simulink model "parallel_phase_voltages_per_switching_state_6"  (R2022a)
settings: Solver=FixedStepDiscrete  StartTime=0.0  StopTime=10.0  RelTol=1e-3
values from neighbouring files (symbols this model uses):
  f_c = 100000    [MPC_params.m]
  Rt = 1e-8    (= 1e-08)    [MPC_params.m]
  u_dc = 565    [MPC_params.m]
libraries: simulink x2, hdlsllib x2
(part 3 of 4)

== matlab function parallel_phase_voltages_per_switching_state_6/Phase_voltages_per_switching_state/Subsystem/MATLAB Function12 ==
  data: theta_el_with_offset input; d_voltage_per_switching_state output; u_dc_link_voltage input; Index input; q_voltage_per_switching_state output; x_voltage_per_switching_state output; y_voltage_per_switching_state output
function [d_voltage_per_switching_state, q_voltage_per_switching_state, x_voltage_per_switching_state, y_voltage_per_switching_state] = fcn(theta_el_with_offset, u_dc_link_voltage, Index)
      
        % Initial condition
            Index = Index+1+12;

    
        % Swichtingstates factors alpha beta x y
        Factors_alpha_beta_x_y = single([0	    0.333333333333333	-0.166666666666667	 0.166666666666667	-0.166666666666667	 0.166666666666667	-0.333333333333333	0	 0.288675134594813	0.622008467928146	 0.122008467928146  	0.455341801261480	 0.122008467928146	 0.455341801261480	-0.0446581987385205  0.288675134594813	-0.288675134594813	0.0446581987385205	-0.455341801261480	-0.122008467928146	-0.455341801261480	-0.122008467928146	-0.622008467928146	-0.288675134594813	0	                0.333333333333333	-0.166666666666667  	0.166666666666667	-0.166666666666667	 0.166666666666667	 -0.333333333333333	0	                 0	                 0.333333333333333	-0.166666666666667	  0.166666666666667	    -0.166666666666667	  0.166666666666667	    -0.333333333333333	 0	                 0.288675134594813	 0.622008467928146	 0.122008467928146	 0.455341801261480	 0.122008467928146	 0.455341801261480	-0.0446581987385205  0.288675134594813	-0.288675134594813	 0.0446581987385205  -0.455341801261480	  -0.122008467928146	-0.455341801261480	-0.122008467928146	-0.622008467928146	-0.288675134594813	0	0.333333333333333	-0.166666666666667	 0.166666666666667	-0.166666666666667	 0.166666666666667	-0.333333333333333	0;
                                         0	    0                    0.288675134594813	 0.288675134594813	-0.288675134594813	-0.288675134594813	 0	                0	 0.166666666666667	0.166666666666667	 0.455341801261480  	0.455341801261480	-0.122008467928146	-0.122008467928146	 0.166666666666667	 0.166666666666667	 0.166666666666667	0.166666666666667	 0.455341801261480   0.455341801261480	-0.122008467928146	-0.122008467928146	 0.166666666666667	 0.166666666666667	0.333333333333333	0.333333333333333	 0.622008467928146	    0.622008467928146	 0.0446581987385205	 0.0446581987385205	  0.333333333333333	0.333333333333333	-0.333333333333333	-0.333333333333333	-0.0446581987385205	 -0.0446581987385205	-0.622008467928146	 -0.622008467928146	    -0.333333333333333	-0.333333333333333	-0.166666666666667	-0.166666666666667	 0.122008467928146	 0.122008467928146	-0.455341801261480	-0.455341801261480	-0.166666666666667	-0.166666666666667	-0.166666666666667	-0.166666666666667	  0.122008467928146	   0.122008467928146	-0.455341801261480	-0.455341801261480	-0.166666666666667	-0.166666666666667	0	0	                 0.288675134594813	 0.288675134594813	-0.288675134594813	-0.288675134594813	 0	                0;
                                         0	    0.333333333333333	-0.166666666666667	 0.166666666666667	-0.166666666666667	 0.166666666666667	-0.333333333333333	0	-0.288675134594813	0.0446581987385205	-0.455341801261480	   -0.122008467928146	-0.455341801261480	-0.122008467928146	-0.622008467928146	-0.288675134594813	 0.288675134594813	0.622008467928146	 0.122008467928146	 0.455341801261480   0.122008467928146	 0.455341801261480	-0.0446581987385205	 0.288675134594813	0	                0.333333333333333	-0.166666666666667	    0.166666666666667	-0.166666666666667	 0.166666666666667	 -0.333333333333333	0	                 0	                 0.333333333333333	-0.166666666666667	  0.166666666666667	    -0.166666666666667	  0.166666666666667	    -0.333333333333333	 0	                -0.288675134594813	 0.0446581987385205	-0.455341801261480	-0.122008467928146	-0.455341801261480	-0.122008467928146	-0.622008467928146	-0.288675134594813	 0.288675134594813	 0.622008467928146	  0.122008467928146	   0.455341801261480	 0.122008467928146	 0.455341801261480	-0.0446581987385205  0.288675134594813	0	0.333333333333333	-0.166666666666667	 0.166666666666667	-0.166666666666667	 0.166666666666667	-0.333333333333333	0;
                                         0	    0	                -0.288675134594813	-0.288675134594813	 0.288675134594813	 0.288675134594813	 0              	0	 0.166666666666667	0.166666666666667	-0.122008467928146     -0.122008467928146	 0.455341801261480	 0.455341801261480	 0.166666666666667	 0.166666666666667	 0.166666666666667	0.166666666666667	-0.122008467928146	-0.122008467928146	 0.455341801261480	 0.455341801261480	 0.166666666666667	 0.166666666666667	0.333333333333333	0.333333333333333	 0.0446581987385205 	0.0446581987385205	 0.622008467928146	 0.622008467928146	  0.333333333333333	0.333333333333333	-0.333333333333333	-0.333333333333333	-0.622008467928146	 -0.622008467928146	    -0.0446581987385205	 -0.0446581987385205	-0.333333333333333	-0.333333333333333	-0.166666666666667	-0.166666666666667	-0.455341801261480	-0.455341801261480	 0.122008467928146	 0.122008467928146	-0.166666666666667	-0.166666666666667	-0.166666666666667	-0.166666666666667	 -0.455341801261480	  -0.455341801261480	 0.122008467928146	 0.122008467928146	-0.166666666666667	-0.166666666666667	0	0	                -0.288675134594813	-0.288675134594813	 0.288675134594813	 0.288675134594813	 0	                0]);
        
        % Park-Transformation of the switchingstates factors
        Factors_d_q_x_y =single(zeros(4,1));
    
        Factors_d_q_x_y(3,1) = Factors_alpha_beta_x_y(3,Index);
        Factors_d_q_x_y(4,1) = Factors_alpha_beta_x_y(4,Index);
    
        cos_theta_el = single(cos(theta_el_with_offset));
        sin_theta_el = single(sin(theta_el_with_offset));
       
        Factors_d_q_x_y(1,1) = cos_theta_el*Factors_alpha_beta_x_y(1,Index)+sin_theta_el*Factors_alpha_beta_x_y(2,Index);
        Factors_d_q_x_y(2,1) = -sin_theta_el*Factors_alpha_beta_x_y(1,Index)+cos_theta_el*Factors_alpha_beta_x_y(2,Index);
    
        %Calculation of the voltages per switching state in alpha beta coordinates
        d_q_x_y_voltages_per_switching_state = single(u_dc_link_voltage*Factors_d_q_x_y);
    
        d_voltage_per_switching_state = d_q_x_y_voltages_per_switching_state(1,1);
        q_voltage_per_switching_state = d_q_x_y_voltages_per_switching_state(2,1);
        x_voltage_per_switching_state = d_q_x_y_voltages_per_switching_state(3,1);
        y_voltage_per_switching_state = d_q_x_y_voltages_per_switching_state(4,1);
    

end

== matlab function parallel_phase_voltages_per_switching_state_6/Phase_voltages_per_switching_state/Subsystem/MATLAB Function13 ==
  data: theta_el_with_offset input; d_voltage_per_switching_state output; u_dc_link_voltage input; Index input; q_voltage_per_switching_state output; x_voltage_per_switching_state output; y_voltage_per_switching_state output
function [d_voltage_per_switching_state, q_voltage_per_switching_state, x_voltage_per_switching_state, y_voltage_per_switching_state] = fcn(theta_el_with_offset, u_dc_link_voltage, Index)
      
        % Initial condition
            Index = Index+1+8;

    
        % Swichtingstates factors alpha beta x y
        Factors_alpha_beta_x_y = single([0	    0.333333333333333	-0.166666666666667	 0.166666666666667	-0.166666666666667	 0.166666666666667	-0.333333333333333	0	 0.288675134594813	0.622008467928146	 0.122008467928146  	0.455341801261480	 0.122008467928146	 0.455341801261480	-0.0446581987385205  0.288675134594813	-0.288675134594813	0.0446581987385205	-0.455341801261480	-0.122008467928146	-0.455341801261480	-0.122008467928146	-0.622008467928146	-0.288675134594813	0	                0.333333333333333	-0.166666666666667  	0.166666666666667	-0.166666666666667	 0.166666666666667	 -0.333333333333333	0	                 0	                 0.333333333333333	-0.166666666666667	  0.166666666666667	    -0.166666666666667	  0.166666666666667	    -0.333333333333333	 0	                 0.288675134594813	 0.622008467928146	 0.122008467928146	 0.455341801261480	 0.122008467928146	 0.455341801261480	-0.0446581987385205  0.288675134594813	-0.288675134594813	 0.0446581987385205  -0.455341801261480	  -0.122008467928146	-0.455341801261480	-0.122008467928146	-0.622008467928146	-0.288675134594813	0	0.333333333333333	-0.166666666666667	 0.166666666666667	-0.166666666666667	 0.166666666666667	-0.333333333333333	0;
                                         0	    0                    0.288675134594813	 0.288675134594813	-0.288675134594813	-0.288675134594813	 0	                0	 0.166666666666667	0.166666666666667	 0.455341801261480  	0.455341801261480	-0.122008467928146	-0.122008467928146	 0.166666666666667	 0.166666666666667	 0.166666666666667	0.166666666666667	 0.455341801261480   0.455341801261480	-0.122008467928146	-0.122008467928146	 0.166666666666667	 0.166666666666667	0.333333333333333	0.333333333333333	 0.622008467928146	    0.622008467928146	 0.0446581987385205	 0.0446581987385205	  0.333333333333333	0.333333333333333	-0.333333333333333	-0.333333333333333	-0.0446581987385205	 -0.0446581987385205	-0.622008467928146	 -0.622008467928146	    -0.333333333333333	-0.333333333333333	-0.166666666666667	-0.166666666666667	 0.122008467928146	 0.122008467928146	-0.455341801261480	-0.455341801261480	-0.166666666666667	-0.166666666666667	-0.166666666666667	-0.166666666666667	  0.122008467928146	   0.122008467928146	-0.455341801261480	-0.455341801261480	-0.166666666666667	-0.166666666666667	0	0	                 0.288675134594813	 0.288675134594813	-0.288675134594813	-0.288675134594813	 0	                0;
                                         0	    0.333333333333333	-0.166666666666667	 0.166666666666667	-0.166666666666667	 0.166666666666667	-0.333333333333333	0	-0.288675134594813	0.0446581987385205	-0.455341801261480	   -0.122008467928146	-0.455341801261480	-0.122008467928146	-0.622008467928146	-0.288675134594813	 0.288675134594813	0.622008467928146	 0.122008467928146	 0.455341801261480   0.122008467928146	 0.455341801261480	-0.0446581987385205	 0.288675134594813	0	                0.333333333333333	-0.166666666666667	    0.166666666666667	-0.166666666666667	 0.166666666666667	 -0.333333333333333	0	                 0	                 0.333333333333333	-0.166666666666667	  0.166666666666667	    -0.166666666666667	  0.166666666666667	    -0.333333333333333	 0	                -0.288675134594813	 0.0446581987385205	-0.455341801261480	-0.122008467928146	-0.455341801261480	-0.122008467928146	-0.622008467928146	-0.288675134594813	 0.288675134594813	 0.622008467928146	  0.122008467928146	   0.455341801261480	 0.122008467928146	 0.455341801261480	-0.0446581987385205  0.288675134594813	0	0.333333333333333	-0.166666666666667	 0.166666666666667	-0.166666666666667	 0.166666666666667	-0.333333333333333	0;
                                         0	    0	                -0.288675134594813	-0.288675134594813	 0.288675134594813	 0.288675134594813	 0              	0	 0.166666666666667	0.166666666666667	-0.122008467928146     -0.122008467928146	 0.455341801261480	 0.455341801261480	 0.166666666666667	 0.166666666666667	 0.166666666666667	0.166666666666667	-0.122008467928146	-0.122008467928146	 0.455341801261480	 0.455341801261480	 0.166666666666667	 0.166666666666667	0.333333333333333	0.333333333333333	 0.0446581987385205 	0.0446581987385205	 0.622008467928146	 0.622008467928146	  0.333333333333333	0.333333333333333	-0.333333333333333	-0.333333333333333	-0.622008467928146	 -0.622008467928146	    -0.0446581987385205	 -0.0446581987385205	-0.333333333333333	-0.333333333333333	-0.166666666666667	-0.166666666666667	-0.455341801261480	-0.455341801261480	 0.122008467928146	 0.122008467928146	-0.166666666666667	-0.166666666666667	-0.166666666666667	-0.166666666666667	 -0.455341801261480	  -0.455341801261480	 0.122008467928146	 0.122008467928146	-0.166666666666667	-0.166666666666667	0	0	                -0.288675134594813	-0.288675134594813	 0.288675134594813	 0.288675134594813	 0	                0]);
        
        % Park-Transformation of the switchingstates factors
        Factors_d_q_x_y =single(zeros(4,1));
    
        Factors_d_q_x_y(3,1) = Factors_alpha_beta_x_y(3,Index);
        Factors_d_q_x_y(4,1) = Factors_alpha_beta_x_y(4,Index);
    
        cos_theta_el = single(cos(theta_el_with_offset));
        sin_theta_el = single(sin(theta_el_with_offset));
       
        Factors_d_q_x_y(1,1) = cos_theta_el*Factors_alpha_beta_x_y(1,Index)+sin_theta_el*Factors_alpha_beta_x_y(2,Index);
        Factors_d_q_x_y(2,1) = -sin_theta_el*Factors_alpha_beta_x_y(1,Index)+cos_theta_el*Factors_alpha_beta_x_y(2,Index);
    
        %Calculation of the voltages per switching state in alpha beta coordinates
        d_q_x_y_voltages_per_switching_state = single(u_dc_link_voltage*Factors_d_q_x_y);
    
        d_voltage_per_switching_state = d_q_x_y_voltages_per_switching_state(1,1);
        q_voltage_per_switching_state = d_q_x_y_voltages_per_switching_state(2,1);
        x_voltage_per_switching_state = d_q_x_y_voltages_per_switching_state(3,1);
        y_voltage_per_switching_state = d_q_x_y_voltages_per_switching_state(4,1);
    

end

== matlab function parallel_phase_voltages_per_switching_state_6/Phase_voltages_per_switching_state/Subsystem/MATLAB Function14 ==
  data: theta_el_with_offset input; d_voltage_per_switching_state output; u_dc_link_voltage input; Index input; q_voltage_per_switching_state output; x_voltage_per_switching_state output; y_voltage_per_switching_state output
function [d_voltage_per_switching_state, q_voltage_per_switching_state, x_voltage_per_switching_state, y_voltage_per_switching_state] = fcn(theta_el_with_offset, u_dc_link_voltage, Index)
      
        % Initial condition
            Index = Index+1+4;

    
        % Swichtingstates factors alpha beta x y
        Factors_alpha_beta_x_y = single([0	    0.333333333333333	-0.166666666666667	 0.166666666666667	-0.166666666666667	 0.166666666666667	-0.333333333333333	0	 0.288675134594813	0.622008467928146	 0.122008467928146  	0.455341801261480	 0.122008467928146	 0.455341801261480	-0.0446581987385205  0.288675134594813	-0.288675134594813	0.0446581987385205	-0.455341801261480	-0.122008467928146	-0.455341801261480	-0.122008467928146	-0.622008467928146	-0.288675134594813	0	                0.333333333333333	-0.166666666666667  	0.166666666666667	-0.166666666666667	 0.166666666666667	 -0.333333333333333	0	                 0	                 0.333333333333333	-0.166666666666667	  0.166666666666667	    -0.166666666666667	  0.166666666666667	    -0.333333333333333	 0	                 0.288675134594813	 0.622008467928146	 0.122008467928146	 0.455341801261480	 0.122008467928146	 0.455341801261480	-0.0446581987385205  0.288675134594813	-0.288675134594813	 0.0446581987385205  -0.455341801261480	  -0.122008467928146	-0.455341801261480	-0.122008467928146	-0.622008467928146	-0.288675134594813	0	0.333333333333333	-0.166666666666667	 0.166666666666667	-0.166666666666667	 0.166666666666667	-0.333333333333333	0;
                                         0	    0                    0.288675134594813	 0.288675134594813	-0.288675134594813	-0.288675134594813	 0	                0	 0.166666666666667	0.166666666666667	 0.455341801261480  	0.455341801261480	-0.122008467928146	-0.122008467928146	 0.166666666666667	 0.166666666666667	 0.166666666666667	0.166666666666667	 0.455341801261480   0.455341801261480	-0.122008467928146	-0.122008467928146	 0.166666666666667	 0.166666666666667	0.333333333333333	0.333333333333333	 0.622008467928146	    0.622008467928146	 0.0446581987385205	 0.0446581987385205	  0.333333333333333	0.333333333333333	-0.333333333333333	-0.333333333333333	-0.0446581987385205	 -0.0446581987385205	-0.622008467928146	 -0.622008467928146	    -0.333333333333333	-0.333333333333333	-0.166666666666667	-0.166666666666667	 0.122008467928146	 0.122008467928146	-0.455341801261480	-0.455341801261480	-0.166666666666667	-0.166666666666667	-0.166666666666667	-0.166666666666667	  0.122008467928146	   0.122008467928146	-0.455341801261480	-0.455341801261480	-0.166666666666667	-0.166666666666667	0	0	                 0.288675134594813	 0.288675134594813	-0.288675134594813	-0.288675134594813	 0	                0;
                                         0	    0.333333333333333	-0.166666666666667	 0.166666666666667	-0.166666666666667	 0.166666666666667	-0.333333333333333	0	-0.288675134594813	0.0446581987385205	-0.455341801261480	   -0.122008467928146	-0.455341801261480	-0.122008467928146	-0.622008467928146	-0.288675134594813	 0.288675134594813	0.622008467928146	 0.122008467928146	 0.455341801261480   0.122008467928146	 0.455341801261480	-0.0446581987385205	 0.288675134594813	0	                0.333333333333333	-0.166666666666667	    0.166666666666667	-0.166666666666667	 0.166666666666667	 -0.333333333333333	0	                 0	                 0.333333333333333	-0.166666666666667	  0.166666666666667	    -0.166666666666667	  0.166666666666667	    -0.333333333333333	 0	                -0.288675134594813	 0.0446581987385205	-0.455341801261480	-0.122008467928146	-0.455341801261480	-0.122008467928146	-0.622008467928146	-0.288675134594813	 0.288675134594813	 0.622008467928146	  0.122008467928146	   0.455341801261480	 0.122008467928146	 0.455341801261480	-0.0446581987385205  0.288675134594813	0	0.333333333333333	-0.166666666666667	 0.166666666666667	-0.166666666666667	 0.166666666666667	-0.333333333333333	0;
                                         0	    0	                -0.288675134594813	-0.288675134594813	 0.288675134594813	 0.288675134594813	 0              	0	 0.166666666666667	0.166666666666667	-0.122008467928146     -0.122008467928146	 0.455341801261480	 0.455341801261480	 0.166666666666667	 0.166666666666667	 0.166666666666667	0.166666666666667	-0.122008467928146	-0.122008467928146	 0.455341801261480	 0.455341801261480	 0.166666666666667	 0.166666666666667	0.333333333333333	0.333333333333333	 0.0446581987385205 	0.0446581987385205	 0.622008467928146	 0.622008467928146	  0.333333333333333	0.333333333333333	-0.333333333333333	-0.333333333333333	-0.622008467928146	 -0.622008467928146	    -0.0446581987385205	 -0.0446581987385205	-0.333333333333333	-0.333333333333333	-0.166666666666667	-0.166666666666667	-0.455341801261480	-0.455341801261480	 0.122008467928146	 0.122008467928146	-0.166666666666667	-0.166666666666667	-0.166666666666667	-0.166666666666667	 -0.455341801261480	  -0.455341801261480	 0.122008467928146	 0.122008467928146	-0.166666666666667	-0.166666666666667	0	0	                -0.288675134594813	-0.288675134594813	 0.288675134594813	 0.288675134594813	 0	                0]);
        
        % Park-Transformation of the switchingstates factors
        Factors_d_q_x_y =single(zeros(4,1));
    
        Factors_d_q_x_y(3,1) = Factors_alpha_beta_x_y(3,Index);
        Factors_d_q_x_y(4,1) = Factors_alpha_beta_x_y(4,Index);
    
        cos_theta_el = single(cos(theta_el_with_offset));
        sin_theta_el = single(sin(theta_el_with_offset));
       
        Factors_d_q_x_y(1,1) = cos_theta_el*Factors_alpha_beta_x_y(1,Index)+sin_theta_el*Factors_alpha_beta_x_y(2,Index);
        Factors_d_q_x_y(2,1) = -sin_theta_el*Factors_alpha_beta_x_y(1,Index)+cos_theta_el*Factors_alpha_beta_x_y(2,Index);
    
        %Calculation of the voltages per switching state in alpha beta coordinates
        d_q_x_y_voltages_per_switching_state = single(u_dc_link_voltage*Factors_d_q_x_y);
    
        d_voltage_per_switching_state = d_q_x_y_voltages_per_switching_state(1,1);
        q_voltage_per_switching_state = d_q_x_y_voltages_per_switching_state(2,1);
        x_voltage_per_switching_state = d_q_x_y_voltages_per_switching_state(3,1);
        y_voltage_per_switching_state = d_q_x_y_voltages_per_switching_state(4,1);
    

end

== matlab function parallel_phase_voltages_per_switching_state_6/Phase_voltages_per_switching_state/Subsystem/MATLAB Function15 ==
  data: theta_el_with_offset input; d_voltage_per_switching_state output; u_dc_link_voltage input; Index input; q_voltage_per_switching_state output; x_voltage_per_switching_state output; y_voltage_per_switching_state output
function [d_voltage_per_switching_state, q_voltage_per_switching_state, x_voltage_per_switching_state, y_voltage_per_switching_state] = fcn(theta_el_with_offset, u_dc_link_voltage, Index)
      
        % Initial condition
            Index = Index+1;

        % Swichtingstates factors alpha beta x y
        Factors_alpha_beta_x_y = single([0	    0.333333333333333	-0.166666666666667	 0.166666666666667	-0.166666666666667	 0.166666666666667	-0.333333333333333	0	 0.288675134594813	0.622008467928146	 0.122008467928146  	0.455341801261480	 0.122008467928146	 0.455341801261480	-0.0446581987385205  0.288675134594813	-0.288675134594813	0.0446581987385205	-0.455341801261480	-0.122008467928146	-0.455341801261480	-0.122008467928146	-0.622008467928146	-0.288675134594813	0	                0.333333333333333	-0.166666666666667  	0.166666666666667	-0.166666666666667	 0.166666666666667	 -0.333333333333333	0	                 0	                 0.333333333333333	-0.166666666666667	  0.166666666666667	    -0.166666666666667	  0.166666666666667	    -0.333333333333333	 0	                 0.288675134594813	 0.622008467928146	 0.122008467928146	 0.455341801261480	 0.122008467928146	 0.455341801261480	-0.0446581987385205  0.288675134594813	-0.288675134594813	 0.0446581987385205  -0.455341801261480	  -0.122008467928146	-0.455341801261480	-0.122008467928146	-0.622008467928146	-0.288675134594813	0	0.333333333333333	-0.166666666666667	 0.166666666666667	-0.166666666666667	 0.166666666666667	-0.333333333333333	0;
                                         0	    0                    0.288675134594813	 0.288675134594813	-0.288675134594813	-0.288675134594813	 0	                0	 0.166666666666667	0.166666666666667	 0.455341801261480  	0.455341801261480	-0.122008467928146	-0.122008467928146	 0.166666666666667	 0.166666666666667	 0.166666666666667	0.166666666666667	 0.455341801261480   0.455341801261480	-0.122008467928146	-0.122008467928146	 0.166666666666667	 0.166666666666667	0.333333333333333	0.333333333333333	 0.622008467928146	    0.622008467928146	 0.0446581987385205	 0.0446581987385205	  0.333333333333333	0.333333333333333	-0.333333333333333	-0.333333333333333	-0.0446581987385205	 -0.0446581987385205	-0.622008467928146	 -0.622008467928146	    -0.333333333333333	-0.333333333333333	-0.166666666666667	-0.166666666666667	 0.122008467928146	 0.122008467928146	-0.455341801261480	-0.455341801261480	-0.166666666666667	-0.166666666666667	-0.166666666666667	-0.166666666666667	  0.122008467928146	   0.122008467928146	-0.455341801261480	-0.455341801261480	-0.166666666666667	-0.166666666666667	0	0	                 0.288675134594813	 0.288675134594813	-0.288675134594813	-0.288675134594813	 0	                0;
                                         0	    0.333333333333333	-0.166666666666667	 0.166666666666667	-0.166666666666667	 0.166666666666667	-0.333333333333333	0	-0.288675134594813	0.0446581987385205	-0.455341801261480	   -0.122008467928146	-0.455341801261480	-0.122008467928146	-0.622008467928146	-0.288675134594813	 0.288675134594813	0.622008467928146	 0.122008467928146	 0.455341801261480   0.122008467928146	 0.455341801261480	-0.0446581987385205	 0.288675134594813	0	                0.333333333333333	-0.166666666666667	    0.166666666666667	-0.166666666666667	 0.166666666666667	 -0.333333333333333	0	                 0	                 0.333333333333333	-0.166666666666667	  0.166666666666667	    -0.166666666666667	  0.166666666666667	    -0.333333333333333	 0	                -0.288675134594813	 0.0446581987385205	-0.455341801261480	-0.122008467928146	-0.455341801261480	-0.122008467928146	-0.622008467928146	-0.288675134594813	 0.288675134594813	 0.622008467928146	  0.122008467928146	   0.455341801261480	 0.122008467928146	 0.455341801261480	-0.0446581987385205  0.288675134594813	0	0.333333333333333	-0.166666666666667	 0.166666666666667	-0.166666666666667	 0.166666666666667	-0.333333333333333	0;
                                         0	    0	                -0.288675134594813	-0.288675134594813	 0.288675134594813	 0.288675134594813	 0              	0	 0.166666666666667	0.166666666666667	-0.122008467928146     -0.122008467928146	 0.455341801261480	 0.455341801261480	 0.166666666666667	 0.166666666666667	 0.166666666666667	0.166666666666667	-0.122008467928146	-0.122008467928146	 0.455341801261480	 0.455341801261480	 0.166666666666667	 0.166666666666667	0.333333333333333	0.333333333333333	 0.0446581987385205 	0.0446581987385205	 0.622008467928146	 0.622008467928146	  0.333333333333333	0.333333333333333	-0.333333333333333	-0.333333333333333	-0.622008467928146	 -0.622008467928146	    -0.0446581987385205	 -0.0446581987385205	-0.333333333333333	-0.333333333333333	-0.166666666666667	-0.166666666666667	-0.455341801261480	-0.455341801261480	 0.122008467928146	 0.122008467928146	-0.166666666666667	-0.166666666666667	-0.166666666666667	-0.166666666666667	 -0.455341801261480	  -0.455341801261480	 0.122008467928146	 0.122008467928146	-0.166666666666667	-0.166666666666667	0	0	                -0.288675134594813	-0.288675134594813	 0.288675134594813	 0.288675134594813	 0	                0]);
        
        % Park-Transformation of the switchingstates factors
        Factors_d_q_x_y =single(zeros(4,1));
    
        Factors_d_q_x_y(3,1) = Factors_alpha_beta_x_y(3,Index);
        Factors_d_q_x_y(4,1) = Factors_alpha_beta_x_y(4,Index);
    
        cos_theta_el = single(cos(theta_el_with_offset));
        sin_theta_el = single(sin(theta_el_with_offset));
       
        Factors_d_q_x_y(1,1) = cos_theta_el*Factors_alpha_beta_x_y(1,Index)+sin_theta_el*Factors_alpha_beta_x_y(2,Index);
        Factors_d_q_x_y(2,1) = -sin_theta_el*Factors_alpha_beta_x_y(1,Index)+cos_theta_el*Factors_alpha_beta_x_y(2,Index);
    
        %Calculation of the voltages per switching state in alpha beta coordinates
        d_q_x_y_voltages_per_switching_state = single(u_dc_link_voltage*Factors_d_q_x_y);
    
        d_voltage_per_switching_state = d_q_x_y_voltages_per_switching_state(1,1);
        q_voltage_per_switching_state = d_q_x_y_voltages_per_switching_state(2,1);
        x_voltage_per_switching_state = d_q_x_y_voltages_per_switching_state(3,1);
        y_voltage_per_switching_state = d_q_x_y_voltages_per_switching_state(4,1);
    

end

== matlab function parallel_phase_voltages_per_switching_state_6/Phase_voltages_per_switching_state/Subsystem/MATLAB Function1 ==
  data: theta_el_with_offset input; d_voltage_per_switching_state output; u_dc_link_voltage input; Index input; q_voltage_per_switching_state output; x_voltage_per_switching_state output; y_voltage_per_switching_state output
function [d_voltage_per_switching_state, q_voltage_per_switching_state, x_voltage_per_switching_state, y_voltage_per_switching_state] = fcn(theta_el_with_offset, u_dc_link_voltage, Index)
      
        % Initial condition
            Index = Index+1+56;

    
        % Swichtingstates factors alpha beta x y
        Factors_alpha_beta_x_y = single([0	    0.333333333333333	-0.166666666666667	 0.166666666666667	-0.166666666666667	 0.166666666666667	-0.333333333333333	0	 0.288675134594813	0.622008467928146	 0.122008467928146  	0.455341801261480	 0.122008467928146	 0.455341801261480	-0.0446581987385205  0.288675134594813	-0.288675134594813	0.0446581987385205	-0.455341801261480	-0.122008467928146	-0.455341801261480	-0.122008467928146	-0.622008467928146	-0.288675134594813	0	                0.333333333333333	-0.166666666666667  	0.166666666666667	-0.166666666666667	 0.166666666666667	 -0.333333333333333	0	                 0	                 0.333333333333333	-0.166666666666667	  0.166666666666667	    -0.166666666666667	  0.166666666666667	    -0.333333333333333	 0	                 0.288675134594813	 0.622008467928146	 0.122008467928146	 0.455341801261480	 0.122008467928146	 0.455341801261480	-0.0446581987385205  0.288675134594813	-0.288675134594813	 0.0446581987385205  -0.455341801261480	  -0.122008467928146	-0.455341801261480	-0.122008467928146	-0.622008467928146	-0.288675134594813	0	0.333333333333333	-0.166666666666667	 0.166666666666667	-0.166666666666667	 0.166666666666667	-0.333333333333333	0;
                                         0	    0                    0.288675134594813	 0.288675134594813	-0.288675134594813	-0.288675134594813	 0	                0	 0.166666666666667	0.166666666666667	 0.455341801261480  	0.455341801261480	-0.122008467928146	-0.122008467928146	 0.166666666666667	 0.166666666666667	 0.166666666666667	0.166666666666667	 0.455341801261480   0.455341801261480	-0.122008467928146	-0.122008467928146	 0.166666666666667	 0.166666666666667	0.333333333333333	0.333333333333333	 0.622008467928146	    0.622008467928146	 0.0446581987385205	 0.0446581987385205	  0.333333333333333	0.333333333333333	-0.333333333333333	-0.333333333333333	-0.0446581987385205	 -0.0446581987385205	-0.622008467928146	 -0.622008467928146	    -0.333333333333333	-0.333333333333333	-0.166666666666667	-0.166666666666667	 0.122008467928146	 0.122008467928146	-0.455341801261480	-0.455341801261480	-0.166666666666667	-0.166666666666667	-0.166666666666667	-0.166666666666667	  0.122008467928146	   0.122008467928146	-0.455341801261480	-0.455341801261480	-0.166666666666667	-0.166666666666667	0	0	                 0.288675134594813	 0.288675134594813	-0.288675134594813	-0.288675134594813	 0	                0;
                                         0	    0.333333333333333	-0.166666666666667	 0.166666666666667	-0.166666666666667	 0.166666666666667	-0.333333333333333	0	-0.288675134594813	0.0446581987385205	-0.455341801261480	   -0.122008467928146	-0.455341801261480	-0.122008467928146	-0.622008467928146	-0.288675134594813	 0.288675134594813	0.622008467928146	 0.122008467928146	 0.455341801261480   0.122008467928146	 0.455341801261480	-0.0446581987385205	 0.288675134594813	0	                0.333333333333333	-0.166666666666667	    0.166666666666667	-0.166666666666667	 0.166666666666667	 -0.333333333333333	0	                 0	                 0.333333333333333	-0.166666666666667	  0.166666666666667	    -0.166666666666667	  0.166666666666667	    -0.333333333333333	 0	                -0.288675134594813	 0.0446581987385205	-0.455341801261480	-0.122008467928146	-0.455341801261480	-0.122008467928146	-0.622008467928146	-0.288675134594813	 0.288675134594813	 0.622008467928146	  0.122008467928146	   0.455341801261480	 0.122008467928146	 0.455341801261480	-0.0446581987385205  0.288675134594813	0	0.333333333333333	-0.166666666666667	 0.166666666666667	-0.166666666666667	 0.166666666666667	-0.333333333333333	0;
                                         0	    0	                -0.288675134594813	-0.288675134594813	 0.288675134594813	 0.288675134594813	 0              	0	 0.166666666666667	0.166666666666667	-0.122008467928146     -0.122008467928146	 0.455341801261480	 0.455341801261480	 0.166666666666667	 0.166666666666667	 0.166666666666667	0.166666666666667	-0.122008467928146	-0.122008467928146	 0.455341801261480	 0.455341801261480	 0.166666666666667	 0.166666666666667	0.333333333333333	0.333333333333333	 0.0446581987385205 	0.0446581987385205	 0.622008467928146	 0.622008467928146	  0.333333333333333	0.333333333333333	-0.333333333333333	-0.333333333333333	-0.622008467928146	 -0.622008467928146	    -0.0446581987385205	 -0.0446581987385205	-0.333333333333333	-0.333333333333333	-0.166666666666667	-0.166666666666667	-0.455341801261480	-0.455341801261480	 0.122008467928146	 0.122008467928146	-0.166666666666667	-0.166666666666667	-0.166666666666667	-0.166666666666667	 -0.455341801261480	  -0.455341801261480	 0.122008467928146	 0.122008467928146	-0.166666666666667	-0.166666666666667	0	0	                -0.288675134594813	-0.288675134594813	 0.288675134594813	 0.288675134594813	 0	                0]);
        
        % Park-Transformation of the switchingstates factors
        Factors_d_q_x_y =single(zeros(4,1));
    
        Factors_d_q_x_y(3,1) = Factors_alpha_beta_x_y(3,Index);
        Factors_d_q_x_y(4,1) = Factors_alpha_beta_x_y(4,Index);
    
        cos_theta_el = single(cos(theta_el_with_offset));
        sin_theta_el = single(sin(theta_el_with_offset));
       
        Factors_d_q_x_y(1,1) = cos_theta_el*Factors_alpha_beta_x_y(1,Index)+sin_theta_el*Factors_alpha_beta_x_y(2,Index);
        Factors_d_q_x_y(2,1) = -sin_theta_el*Factors_alpha_beta_x_y(1,Index)+cos_theta_el*Factors_alpha_beta_x_y(2,Index);
    
        %Calculation of the voltages per switching state in alpha beta coordinates
        d_q_x_y_voltages_per_switching_state = single(u_dc_link_voltage*Factors_d_q_x_y);
    
        d_voltage_per_switching_state = d_q_x_y_voltages_per_switching_state(1,1);
        q_voltage_per_switching_state = d_q_x_y_voltages_per_switching_state(2,1);
        x_voltage_per_switching_state = d_q_x_y_voltages_per_switching_state(3,1);
        y_voltage_per_switching_state = d_q_x_y_voltages_per_switching_state(4,1);
    

end

== matlab function parallel_phase_voltages_per_switching_state_6/Phase_voltages_per_switching_state/Subsystem/MATLAB Function2 ==
  data: theta_el_with_offset input; d_voltage_per_switching_state output; u_dc_link_voltage input; Index input; q_voltage_per_switching_state output; x_voltage_per_switching_state output; y_voltage_per_switching_state output
function [d_voltage_per_switching_state, q_voltage_per_switching_state, x_voltage_per_switching_state, y_voltage_per_switching_state] = fcn(theta_el_with_offset, u_dc_link_voltage, Index)
      
        % Initial condition
            Index = Index+1+52;

        % Swichtingstates factors alpha beta x y
        Factors_alpha_beta_x_y = single([0	    0.333333333333333	-0.166666666666667	 0.166666666666667	-0.166666666666667	 0.166666666666667	-0.333333333333333	0	 0.288675134594813	0.622008467928146	 0.122008467928146  	0.455341801261480	 0.122008467928146	 0.455341801261480	-0.0446581987385205  0.288675134594813	-0.288675134594813	0.0446581987385205	-0.455341801261480	-0.122008467928146	-0.455341801261480	-0.122008467928146	-0.622008467928146	-0.288675134594813	0	                0.333333333333333	-0.166666666666667  	0.166666666666667	-0.166666666666667	 0.166666666666667	 -0.333333333333333	0	                 0	                 0.333333333333333	-0.166666666666667	  0.166666666666667	    -0.166666666666667	  0.166666666666667	    -0.333333333333333	 0	                 0.288675134594813	 0.622008467928146	 0.122008467928146	 0.455341801261480	 0.122008467928146	 0.455341801261480	-0.0446581987385205  0.288675134594813	-0.288675134594813	 0.0446581987385205  -0.455341801261480	  -0.122008467928146	-0.455341801261480	-0.122008467928146	-0.622008467928146	-0.288675134594813	0	0.333333333333333	-0.166666666666667	 0.166666666666667	-0.166666666666667	 0.166666666666667	-0.333333333333333	0;
                                         0	    0                    0.288675134594813	 0.288675134594813	-0.288675134594813	-0.288675134594813	 0	                0	 0.166666666666667	0.166666666666667	 0.455341801261480  	0.455341801261480	-0.122008467928146	-0.122008467928146	 0.166666666666667	 0.166666666666667	 0.166666666666667	0.166666666666667	 0.455341801261480   0.455341801261480	-0.122008467928146	-0.122008467928146	 0.166666666666667	 0.166666666666667	0.333333333333333	0.333333333333333	 0.622008467928146	    0.622008467928146	 0.0446581987385205	 0.0446581987385205	  0.333333333333333	0.333333333333333	-0.333333333333333	-0.333333333333333	-0.0446581987385205	 -0.0446581987385205	-0.622008467928146	 -0.622008467928146	    -0.333333333333333	-0.333333333333333	-0.166666666666667	-0.166666666666667	 0.122008467928146	 0.122008467928146	-0.455341801261480	-0.455341801261480	-0.166666666666667	-0.166666666666667	-0.166666666666667	-0.166666666666667	  0.122008467928146	   0.122008467928146	-0.455341801261480	-0.455341801261480	-0.166666666666667	-0.166666666666667	0	0	                 0.288675134594813	 0.288675134594813	-0.288675134594813	-0.288675134594813	 0	                0;
                                         0	    0.333333333333333	-0.166666666666667	 0.166666666666667	-0.166666666666667	 0.166666666666667	-0.333333333333333	0	-0.288675134594813	0.0446581987385205	-0.455341801261480	   -0.122008467928146	-0.455341801261480	-0.122008467928146	-0.622008467928146	-0.288675134594813	 0.288675134594813	0.622008467928146	 0.122008467928146	 0.455341801261480   0.122008467928146	 0.455341801261480	-0.0446581987385205	 0.288675134594813	0	                0.333333333333333	-0.166666666666667	    0.166666666666667	-0.166666666666667	 0.166666666666667	 -0.333333333333333	0	                 0	                 0.333333333333333	-0.166666666666667	  0.166666666666667	    -0.166666666666667	  0.166666666666667	    -0.333333333333333	 0	                -0.288675134594813	 0.0446581987385205	-0.455341801261480	-0.122008467928146	-0.455341801261480	-0.122008467928146	-0.622008467928146	-0.288675134594813	 0.288675134594813	 0.622008467928146	  0.122008467928146	   0.455341801261480	 0.122008467928146	 0.455341801261480	-0.0446581987385205  0.288675134594813	0	0.333333333333333	-0.166666666666667	 0.166666666666667	-0.166666666666667	 0.166666666666667	-0.333333333333333	0;
                                         0	    0	                -0.288675134594813	-0.288675134594813	 0.288675134594813	 0.288675134594813	 0              	0	 0.166666666666667	0.166666666666667	-0.122008467928146     -0.122008467928146	 0.455341801261480	 0.455341801261480	 0.166666666666667	 0.166666666666667	 0.166666666666667	0.166666666666667	-0.122008467928146	-0.122008467928146	 0.455341801261480	 0.455341801261480	 0.166666666666667	 0.166666666666667	0.333333333333333	0.333333333333333	 0.0446581987385205 	0.0446581987385205	 0.622008467928146	 0.622008467928146	  0.333333333333333	0.333333333333333	-0.333333333333333	-0.333333333333333	-0.622008467928146	 -0.622008467928146	    -0.0446581987385205	 -0.0446581987385205	-0.333333333333333	-0.333333333333333	-0.166666666666667	-0.166666666666667	-0.455341801261480	-0.455341801261480	 0.122008467928146	 0.122008467928146	-0.166666666666667	-0.166666666666667	-0.166666666666667	-0.166666666666667	 -0.455341801261480	  -0.455341801261480	 0.122008467928146	 0.122008467928146	-0.166666666666667	-0.166666666666667	0	0	                -0.288675134594813	-0.288675134594813	 0.288675134594813	 0.288675134594813	 0	                0]);
        
        % Park-Transformation of the switchingstates factors
        Factors_d_q_x_y =single(zeros(4,1));
    
        Factors_d_q_x_y(3,1) = Factors_alpha_beta_x_y(3,Index);
        Factors_d_q_x_y(4,1) = Factors_alpha_beta_x_y(4,Index);
    
        cos_theta_el = single(cos(theta_el_with_offset));
        sin_theta_el = single(sin(theta_el_with_offset));
       
        Factors_d_q_x_y(1,1) = cos_theta_el*Factors_alpha_beta_x_y(1,Index)+sin_theta_el*Factors_alpha_beta_x_y(2,Index);
        Factors_d_q_x_y(2,1) = -sin_theta_el*Factors_alpha_beta_x_y(1,Index)+cos_theta_el*Factors_alpha_beta_x_y(2,Index);
    
        %Calculation of the voltages per switching state in alpha beta coordinates
        d_q_x_y_voltages_per_switching_state = single(u_dc_link_voltage*Factors_d_q_x_y);
    
        d_voltage_per_switching_state = d_q_x_y_voltages_per_switching_state(1,1);
        q_voltage_per_switching_state = d_q_x_y_voltages_per_switching_state(2,1);
        x_voltage_per_switching_state = d_q_x_y_voltages_per_switching_state(3,1);
        y_voltage_per_switching_state = d_q_x_y_voltages_per_switching_state(4,1);
    

end

== matlab function parallel_phase_voltages_per_switching_state_6/Phase_voltages_per_switching_state/Subsystem/MATLAB Function3 ==
  data: theta_el_with_offset input; d_voltage_per_switching_state output; u_dc_link_voltage input; Index input; q_voltage_per_switching_state output; x_voltage_per_switching_state output; y_voltage_per_switching_state output
function [d_voltage_per_switching_state, q_voltage_per_switching_state, x_voltage_per_switching_state, y_voltage_per_switching_state] = fcn(theta_el_with_offset, u_dc_link_voltage, Index)
      
        % Initial condition
            Index = Index+1+48;

    
        % Swichtingstates factors alpha beta x y
        Factors_alpha_beta_x_y = single([0	    0.333333333333333	-0.166666666666667	 0.166666666666667	-0.166666666666667	 0.166666666666667	-0.333333333333333	0	 0.288675134594813	0.622008467928146	 0.122008467928146  	0.455341801261480	 0.122008467928146	 0.455341801261480	-0.0446581987385205  0.288675134594813	-0.288675134594813	0.0446581987385205	-0.455341801261480	-0.122008467928146	-0.455341801261480	-0.122008467928146	-0.622008467928146	-0.288675134594813	0	                0.333333333333333	-0.166666666666667  	0.166666666666667	-0.166666666666667	 0.166666666666667	 -0.333333333333333	0	                 0	                 0.333333333333333	-0.166666666666667	  0.166666666666667	    -0.166666666666667	  0.166666666666667	    -0.333333333333333	 0	                 0.288675134594813	 0.622008467928146	 0.122008467928146	 0.455341801261480	 0.122008467928146	 0.455341801261480	-0.0446581987385205  0.288675134594813	-0.288675134594813	 0.0446581987385205  -0.455341801261480	  -0.122008467928146	-0.455341801261480	-0.122008467928146	-0.622008467928146	-0.288675134594813	0	0.333333333333333	-0.166666666666667	 0.166666666666667	-0.166666666666667	 0.166666666666667	-0.333333333333333	0;
                                         0	    0                    0.288675134594813	 0.288675134594813	-0.288675134594813	-0.288675134594813	 0	                0	 0.166666666666667	0.166666666666667	 0.455341801261480  	0.455341801261480	-0.122008467928146	-0.122008467928146	 0.166666666666667	 0.166666666666667	 0.166666666666667	0.166666666666667	 0.455341801261480   0.455341801261480	-0.122008467928146	-0.122008467928146	 0.166666666666667	 0.166666666666667	0.333333333333333	0.333333333333333	 0.622008467928146	    0.622008467928146	 0.0446581987385205	 0.0446581987385205	  0.333333333333333	0.333333333333333	-0.333333333333333	-0.333333333333333	-0.0446581987385205	 -0.0446581987385205	-0.622008467928146	 -0.622008467928146	    -0.333333333333333	-0.333333333333333	-0.166666666666667	-0.166666666666667	 0.122008467928146	 0.122008467928146	-0.455341801261480	-0.455341801261480	-0.166666666666667	-0.166666666666667	-0.166666666666667	-0.166666666666667	  0.122008467928146	   0.122008467928146	-0.455341801261480	-0.455341801261480	-0.166666666666667	-0.166666666666667	0	0	                 0.288675134594813	 0.288675134594813	-0.288675134594813	-0.288675134594813	 0	                0;
                                         0	    0.333333333333333	-0.166666666666667	 0.166666666666667	-0.166666666666667	 0.166666666666667	-0.333333333333333	0	-0.288675134594813	0.0446581987385205	-0.455341801261480	   -0.122008467928146	-0.455341801261480	-0.122008467928146	-0.622008467928146	-0.288675134594813	 0.288675134594813	0.622008467928146	 0.122008467928146	 0.455341801261480   0.122008467928146	 0.455341801261480	-0.0446581987385205	 0.288675134594813	0	                0.333333333333333	-0.166666666666667	    0.166666666666667	-0.166666666666667	 0.166666666666667	 -0.333333333333333	0	                 0	                 0.333333333333333	-0.166666666666667	  0.166666666666667	    -0.166666666666667	  0.166666666666667	    -0.333333333333333	 0	                -0.288675134594813	 0.0446581987385205	-0.455341801261480	-0.122008467928146	-0.455341801261480	-0.122008467928146	-0.622008467928146	-0.288675134594813	 0.288675134594813	 0.622008467928146	  0.122008467928146	   0.455341801261480	 0.122008467928146	 0.455341801261480	-0.0446581987385205  0.288675134594813	0	0.333333333333333	-0.166666666666667	 0.166666666666667	-0.166666666666667	 0.166666666666667	-0.333333333333333	0;
                                         0	    0	                -0.288675134594813	-0.288675134594813	 0.288675134594813	 0.288675134594813	 0              	0	 0.166666666666667	0.166666666666667	-0.122008467928146     -0.122008467928146	 0.455341801261480	 0.455341801261480	 0.166666666666667	 0.166666666666667	 0.166666666666667	0.166666666666667	-0.122008467928146	-0.122008467928146	 0.455341801261480	 0.455341801261480	 0.166666666666667	 0.166666666666667	0.333333333333333	0.333333333333333	 0.0446581987385205 	0.0446581987385205	 0.622008467928146	 0.622008467928146	  0.333333333333333	0.333333333333333	-0.333333333333333	-0.333333333333333	-0.622008467928146	 -0.622008467928146	    -0.0446581987385205	 -0.0446581987385205	-0.333333333333333	-0.333333333333333	-0.166666666666667	-0.166666666666667	-0.455341801261480	-0.455341801261480	 0.122008467928146	 0.122008467928146	-0.166666666666667	-0.166666666666667	-0.166666666666667	-0.166666666666667	 -0.455341801261480	  -0.455341801261480	 0.122008467928146	 0.122008467928146	-0.166666666666667	-0.166666666666667	0	0	                -0.288675134594813	-0.288675134594813	 0.288675134594813	 0.288675134594813	 0	                0]);
        
        % Park-Transformation of the switchingstates factors
        Factors_d_q_x_y =single(zeros(4,1));
    
        Factors_d_q_x_y(3,1) = Factors_alpha_beta_x_y(3,Index);
        Factors_d_q_x_y(4,1) = Factors_alpha_beta_x_y(4,Index);
    
        cos_theta_el = single(cos(theta_el_with_offset));
        sin_theta_el = single(sin(theta_el_with_offset));
       
        Factors_d_q_x_y(1,1) = cos_theta_el*Factors_alpha_beta_x_y(1,Index)+sin_theta_el*Factors_alpha_beta_x_y(2,Index);
        Factors_d_q_x_y(2,1) = -sin_theta_el*Factors_alpha_beta_x_y(1,Index)+cos_theta_el*Factors_alpha_beta_x_y(2,Index);
    
        %Calculation of the voltages per switching state in alpha beta coordinates
        d_q_x_y_voltages_per_switching_state = single(u_dc_link_voltage*Factors_d_q_x_y);
    
        d_voltage_per_switching_state = d_q_x_y_voltages_per_switching_state(1,1);
        q_voltage_per_switching_state = d_q_x_y_voltages_per_switching_state(2,1);
        x_voltage_per_switching_state = d_q_x_y_voltages_per_switching_state(3,1);
        y_voltage_per_switching_state = d_q_x_y_voltages_per_switching_state(4,1);
    

end
